simulink model "Abs"  (R2020a)
settings: Solver=VariableStepAuto  StartTime=0.0  StopTime=10.0  RelTol=1e-3
settings Model: Creator=royde  LastModifiedBy=royde

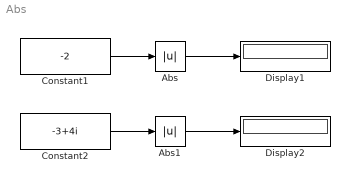
== system Abs ==
  Abs : Abs
  Abs1 : Abs
  Constant1 : Constant  Value=-2
  Constant2 : Constant  Value=-3+4i
  Display1 : Display
  Display2 : Display
  wires:
  Constant1/1 -> Abs/1
  Abs/1 -> Display1/1
  Abs1/1 -> Display2/1
  Constant2/1 -> Abs1/1
